simulink model "HIL_model"  (R2020a)
settings: Solver=ode4  StartTime=0.0  StopTime=inf  FixedStep=0.01  RelTol=1e-3
InitFcn:
  | Init_control
values from neighbouring files (symbols this model uses):
  layer1 = double(results{1,1}.layer9)    [load_parameter.m]
  layer2 = double(results{1,1}.layer10)    [load_parameter.m]
  layer3 = double(results{1,1}.layer11)    [load_parameter.m]
  layer4 = double(results{1,1}.layer12)    [load_parameter.m]
  layer5 = double(results{1,1}.layer13)    [load_parameter.m]
  layer6 = double(results{1,1}.layer14)    [load_parameter.m]
  std = sqrt(max(a,0.01))    [load_parameter.m]
undefined symbols (not defined in the file or in its folder): KiPitchAttitude, KiRollAttitude, Kp_RP_ANGLE, MAX_CONTROL_ANGLE_RATE_Y, MAX_CONTROL_ANGLE_RP
libraries: simulink x3, pixhawk_slib_uORB_RW x2, pixhawk_slib_sensors_actuators x2
settings Model: Creator=Steve  LastModifiedBy=NEW
settings SolverCC: AutoInsertRateTranBlk=on
settings DataIOCC: LimitDataPoints=on  SaveFormat=Array  ReturnWorkspaceOutputs=off
settings OptimizationCC: DefaultParameterBehavior=Inlined  LifeSpan=1  MaxStackSize=64  EfficientTunableParamExpr=on
settings DebuggingCC: SolverPrmCheckMsg=warning  AllowSymbolicDim=off  SFUnexpectedBacktrackingDiag=warning  SFNoUnconditionalDefaultTransitionDiag=warning  SFExecutionAtInitializationDiag=none  ArithmeticOperatorsInVariantConditions=warning
settings HardwareCC: ProdBitPerPointer=32  ProdBitPerSizeT=32  ProdBitPerPtrDiffT=32  ProdLargestAtomicInteger=Long  ProdLargestAtomicFloat=Double  ProdWordSize=32  ProdHWDeviceType=ARM Compatible->ARM Cortex
settings ModelReferenceCC: PropagateSignalLabelsOutOfModel=off
settings SFSimCC: SimUseLocalCustomCode=off  MATLABDynamicMemAlloc=off  CustomCodeUndefinedFunction=UseInterfaceOnly
settings RTWCC: SystemTargetFile=ert.tlc  HardwareBoard=Pixhawk PX4  TemplateMakefile=ert_default_tmf  GenerateReport=on  RTWUseLocalCustomCode=off  Toolchain=Pixhawk Toolchain  IncludeHyperlinkInReport=on  LaunchReport=on  GenerateTraceReport=on  GenerateTraceReportSl=on  GenerateTraceReportSf=on  GenerateTraceReportEml=on  GenerateCodeMetricsReport=on
settings CodeAppCC: IgnoreCustomStorageClasses=off  StateflowObjectComments=on
settings ERTTargetCC: CodeReplacementLibrary=GCC ARM Cortex-A9  MultiwordLength=2048  ExtModeTransport=1  ExtModeMexFile=ext_serial_win32_comm  ExtModeMexArgs=/dev/serial  ERTCustomFileTemplate=PX4_codertarget_file_process.tlc  ConvertIfToSwitch=off  SuppressUnreachableDefaultCases=off
settings ConfigComp: CovMetricSettings=dw  CovHtmlReporting=on  CovSaveCumulativeToWorkspaceVar=on  CovSaveSingleToWorkspaceVar=on  CovExternalEMLEnable=off  CovSFcnEnable=off

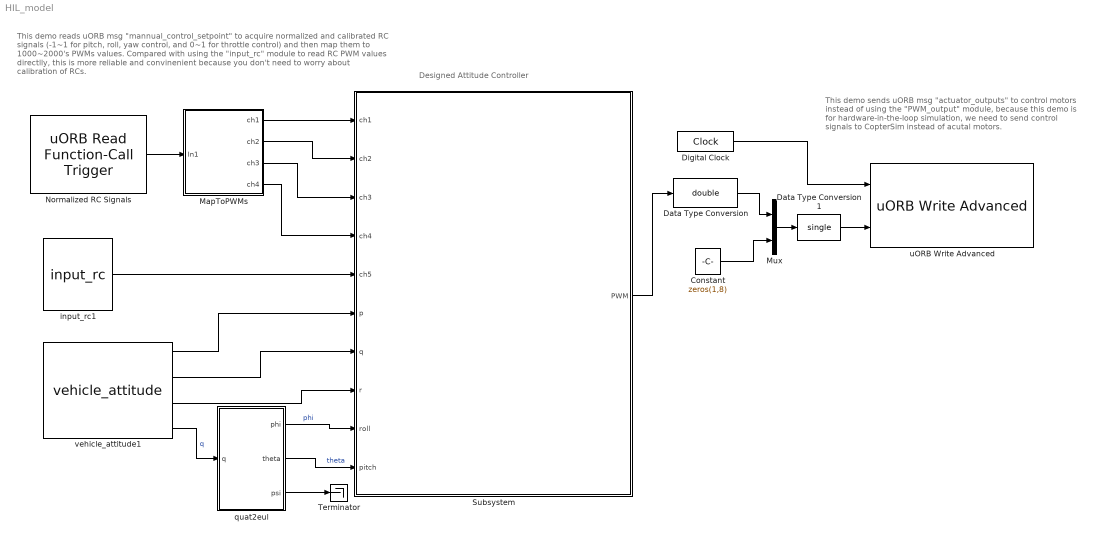
== system HIL_model ==
  note: Designed Attitude Controller
  note: This demo reads uORB msg "mannual_control_setpoint" to acquire normalized and calibrated RC signals (-1~1 for pitch, roll, yaw control, and 0~1 for throttle control) and then map them to 1000~2000's PWMs values.
      | Compared with using the "input_rc" module to read RC PWM values directlly, this is more reliable and convinenient because you don't need to worry about calibration of RCs.
  note: This demo sends uORB msg "actuator_outputs" to control motors instead of using the "PWM_output" module, because this demo is for hardware-in-the-loop simulation, we need to send control signals to CopterSim instead of acutal motors.
  Constant : Constant  Value=zeros(1,8)
  Data Type Conversion : DataTypeConversion  OutDataTypeStr=double
  Data Type Conversion1 : DataTypeConversion  OutDataTypeStr=single
  Digital Clock : DigitalClock  SampleTime=-1
  MapToPWMs : Subsystem
  Mux : Mux  Inputs=2
  Normalized RC Signals : pixhawk_slib_uORB_RW/uORB Read Function-Call Trigger  uORB_Topic_str='manual_control_setpoint'  BusObjVar=Bus: manual_control_setpoint_SL  uORB_Interval=1  AsyncOutput=off  Fcn_call_select=Generate Function Call Signal  TaskName='Task1'  Poll_timeout=100  Ts=-1
      settings: SourceProductName=Pixhawk Target Blocks
  Subsystem : Subsystem
      mask Display: image('./icon/pixhawk.png');
  Terminator : Terminator
  input_rc1 : pixhawk_slib_sensors_actuators/input_rc  Description=|  sampletime=-1  channel1=off  channel2=off  channel3=off  channel4=off  channel5=on  channel6=off  channel7=off  channel8=off  channel9=off  channel10=off  channel11=off  channel12=off  channel13=off  channel14=off  channel15=off  channel16=off  channel17=off  channel18=off  ch_count=off  rssi=off  rc_failsafe=off  rc_lost=off  rc_inputsource=off
      | RC Input Block
      | 
      | This block provides user input control to the model.
      | It uses the input_rc uORB topic.
      | 
      | The user has the ability to choose which channels are available as outputs from this block and also some optional outputs. These include 
      | Channels 1 through 18
      | double data type indicating the PWM value from the controller 
      | measured pulse widths for each of the supported channels 
      | Channel Count 
      | uint32 data type of the number of channels which are detector by the PX4 
      | RC Failsafe 
      | boolean data types indicating that the RC Tx is sending the FailSafe signal (if equipped and properly setup) 
      | explicit failsafe flag: true on TX failure or TX out of range , false otherwise. 
      | Only the true state is reliable, as there are some (PPM) receivers on the market going into failsafe without telling us explicitly. 
      | RC Input Source 
      | Enumeration data type indicating which source the RC input is from. 
      | Valid values are found in the ENUM file: RC_INPUT_SOURCE_ENUM.m 
      |           Enumeration members for class 'RC_INPUT_SOURCE_ENUM':
      |           RCINPUT_SOURCE_UNKNOWN         (0)
      |           RCINPUT_SOURCE_PX4FMU_PPM      (1)
      |           RCINPUT_SOURCE_PX4IO_PPM       (2)
      |           RCINPUT_SOURCE_PX4IO_SPEKTRUM  (3)
      |           RCINPUT_SOURCE_PX4IO_SBUS      (4)
      |           RCINPUT_SOURCE_PX4IO_ST24      (5)
      |           RCINPUT_SOURCE_MAVLINK         (6)
      |           RCINPUT_SOURCE_QURT            (7)
      |           RCINPUT_SOURCE_PX4FMU_SPEKTRUM (8)
      |           RCINPUT_SOURCE_PX4FMU_SBUS     (9)
      |           RCINPUT_SOURCE_PX4FMU_ST24     (10)
      |           RCINPUT_SOURCE_PX4FMU_SUMD     (11)
      |           RCINPUT_SOURCE_PX4FMU_DSM      (12)
      |           RCINPUT_SOURCE_PX4IO_SUMD      (13)
      | 
      | RSSI - Receive signal strength index 
      | receive signal strength indicator (RSSI): < 0: Undefined, 0: no signal, 255: full reception 
      | RC Lost Connection 
      | boolean data type indicating RC receiver connection status 
      | True, if no frame has arrived in the expected time, false otherwise. 
      | True usally means that the receiver has been disconnected, but can also indicate a radio link loss on "stupid" systems. 
      | Will remain false, if a RX with failsafe option continues to transmit frames after a link loss. 
      |   
      | Sample Model: px4demo_input_rc.slx
      settings: SourceProductName=Pixhawk Target Blocks
  quat2eul : MATLAB Function  TreatAsAtomicUnit=on
  uORB Write Advanced : pixhawk_slib_uORB_RW/uORB Write Advanced  Ts=0  uORB_AdvtQueue=on  uORB_FieldEnabledArr="0  0  0  1  0  0  0  0  0  0  0"  uORB_Topic_str=0  uORB_Struct_DT="[1  1  1  1  1]"  BlockInputCount=5  uORB_StructParams="[\"voltage_v\",\"voltage_filtered_v\",\"current_a\",\"current_filtered_a\",\"remaining\"]"  uORB_PortSizes="[1  1  1  1]"  MsgSizeOf=0  MW_update=true
      settings: SourceProductName=Pixhawk Target Blocks
  vehicle_attitude1 : pixhawk_slib_sensors_actuators/vehicle_attitude  sampletime=-1  show_r=on  show_p=on  show_y=on  show_q=on  show_ts=off
      settings: SourceProductName=Pixhawk Target Blocks
  wires:
  quat2eul/1(phi) -> Subsystem/9(roll)  "phi"
  quat2eul/2(theta) -> Subsystem/10(pitch)  "theta"
  vehicle_attitude1/1 -> Subsystem/6(p)
  vehicle_attitude1/2 -> Subsystem/7(q)
  vehicle_attitude1/3 -> Subsystem/8(r)
  Digital Clock/1 -> uORB Write Advanced/1
  Subsystem/1(PWM) -> Data Type Conversion/1
  Constant/1 -> Mux/2
  Mux/1 -> Data Type Conversion1/1
  Data Type Conversion/1 -> Mux/1
  vehicle_attitude1/4 -> quat2eul/1(q)  "q"
  quat2eul/3(psi) -> Terminator/1
  Data Type Conversion1/1 -> uORB Write Advanced/2
  input_rc1/1 -> Subsystem/5(ch5)
  MapToPWMs/4(ch4) -> Subsystem/4(ch4)
  MapToPWMs/3(ch3) -> Subsystem/3(ch3)
  Normalized RC Signals/1 -> MapToPWMs/1(In1)
  MapToPWMs/1(ch1) -> Subsystem/1(ch1)
  MapToPWMs/2(ch2) -> Subsystem/2(ch2)

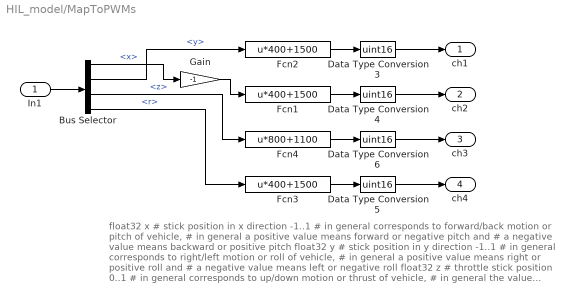
== system HIL_model/MapToPWMs ==
  note: float32 x			 # stick position in x direction -1..1
      | 				 # in general corresponds to forward/back motion or pitch of vehicle,
      | 				 # in general a positive value means forward or negative pitch and
      | 				 # a negative value means backward or positive pitch
      | float32 y			 # stick position in y direction -1..1
      | 				 # in general corresponds to right/left motion or roll of vehicle,
      | 				 # in general a positive value means right or positive roll and
      | 				 # a negative value means left or negative roll
      | float32 z			 # throttle stick position 0..1
      | 				 # in general corresponds to up/down motion or thrust of vehicle,
      | 				 # in general the value corresponds to the demanded throttle by the user,
      | 				 # if the input is used for setting the setpoint of a vertical position
      | 				 # controller any value > 0.5 means up and any value < 0.5 means down
      | float32 r			 # yaw stick/twist position, -1..1
      | 				 # in general corresponds to the righthand rotation around the vertical
      | 				 # (downwards) axis of the vehicle
  In1 : Inport
  Bus Selector : BusSelector  OutputSignals=x,y,z,r
  Data Type Conversion{3..6} (4 alike) : DataTypeConversion  OutDataTypeStr=uint16
  Fcn1 : Fcn  Expr=u*400+1500
  Fcn2 : Fcn  Expr=u*400+1500
  Fcn3 : Fcn  Expr=u*400+1500
  Fcn4 : Fcn  Expr=u*800+1100
  Gain : Gain  Gain=-1
  ch1 : Outport  VectorParamsAs1DForOutWhenUnconnected=off
  ch2 : Outport  Port=2  VectorParamsAs1DForOutWhenUnconnected=off
  ch3 : Outport  Port=3  VectorParamsAs1DForOutWhenUnconnected=off
  ch4 : Outport  Port=4  VectorParamsAs1DForOutWhenUnconnected=off
  wires:
  Bus Selector/2 -> Fcn2/1  "<y>"
  Fcn2/1 -> Data Type Conversion3/1
  Bus Selector/1 -> Gain/1  "<x>"
  In1/1 -> Bus Selector/1
  Bus Selector/3 -> Fcn4/1  "<z>"
  Fcn1/1 -> Data Type Conversion4/1
  Bus Selector/4 -> Fcn3/1  "<r>"
  Data Type Conversion4/1 -> ch2/1
  Data Type Conversion5/1 -> ch4/1
  Data Type Conversion6/1 -> ch3/1
  Fcn4/1 -> Data Type Conversion6/1
  Fcn3/1 -> Data Type Conversion5/1
  Data Type Conversion3/1 -> ch1/1
  Gain/1 -> Fcn1/1

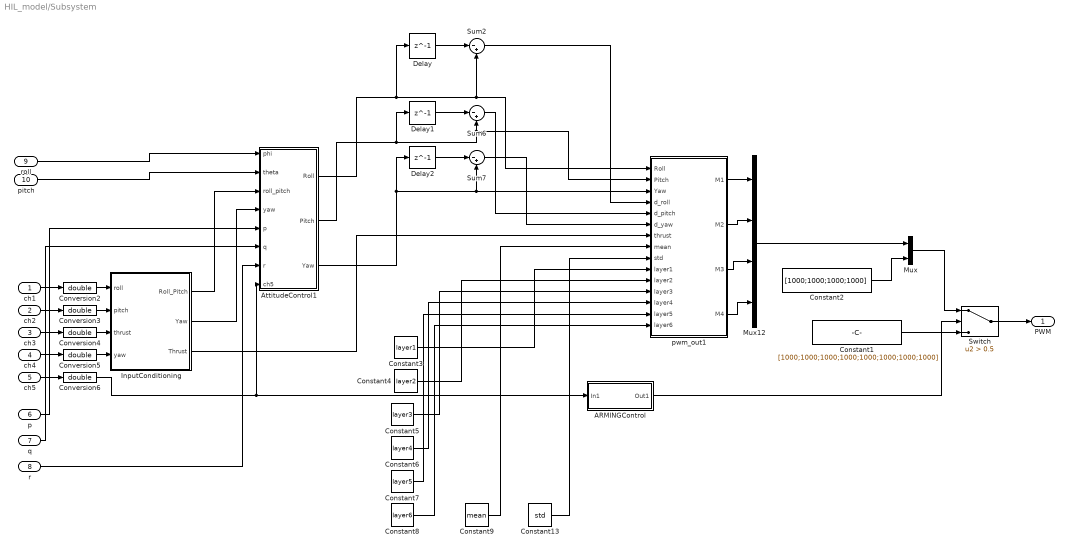
== system HIL_model/Subsystem ==
  ch1 : Inport  OutDataTypeStr=uint16  PortDimensions=1
  ch2 : Inport  Port=2  OutDataTypeStr=uint16  PortDimensions=1
  ch3 : Inport  Port=3  OutDataTypeStr=uint16  PortDimensions=1
  ch4 : Inport  Port=4  OutDataTypeStr=uint16  PortDimensions=1
  ch5 : Inport  Port=5  OutDataTypeStr=uint16  PortDimensions=1  Interpolate=off
  p : Inport  Port=6  PortDimensions=1
  q : Inport  Port=7  PortDimensions=1
  r : Inport  Port=8  PortDimensions=1
  roll : Inport  Port=9  PortDimensions=1
  pitch : Inport  Port=10  PortDimensions=1
  ARMINGControl : Subsystem
  AttitudeControl1 : Subsystem
  Constant1 : Constant  Value=[1000;1000;1000;1000;1000;1000;1000;1000]
  Constant13 : Constant  Value=std
  Constant2 : Constant  Value=[1000;1000;1000;1000]
  Constant3 : Constant  Value=layer1
  Constant4 : Constant  Value=layer2
  Constant5 : Constant  Value=layer3
  Constant6 : Constant  Value=layer4
  Constant7 : Constant  Value=layer5
  Constant8 : Constant  Value=layer6
  Constant9 : Constant  Value=mean
  Conversion{2..6} (5 alike) : DataTypeConversion  OutDataTypeStr=double
  Delay : Delay  DelayLength=1  InitialCondition=0
  Delay1 : Delay  DelayLength=1  InitialCondition=0
  Delay2 : Delay  DelayLength=1  InitialCondition=0
  InputConditioning : Subsystem
  Mux : Mux  Inputs=2
  Mux12 : Mux
  Sum2 : Sum  Inputs=|-+
  Sum6 : Sum  Inputs=|-+
  Sum7 : Sum  Inputs=|-+
  Switch : Switch  Criteria=u2 > Threshold  Threshold=0.5
  pwm_out1 : MATLAB Function  TreatAsAtomicUnit=on
  PWM : Outport  PortDimensions=8  VectorParamsAs1DForOutWhenUnconnected=off
  wires:
  InputConditioning/3(Thrust) -> pwm_out1/7(thrust)
  q/1 -> AttitudeControl1/6(q)
  ARMINGControl/1(Out1) -> Switch/2
  pitch/1 -> AttitudeControl1/2(theta)
  Conversion5/1 -> InputConditioning/4(yaw)
  Mux12/1 -> Mux/1
  pwm_out1/1(M1) -> Mux12/1
  pwm_out1/2(M2) -> Mux12/2
  ch4/1 -> Conversion5/1
  r/1 -> AttitudeControl1/7(r)
  ch2/1 -> Conversion3/1
  ch5/1 -> Conversion6/1
  roll/1 -> AttitudeControl1/1(phi)
  Conversion3/1 -> InputConditioning/2(pitch)
  Conversion4/1 -> InputConditioning/3(thrust)
  Conversion6/1 -> AttitudeControl1/8(ch5), ARMINGControl/1(In1)
  Conversion2/1 -> InputConditioning/1(roll)
  ch1/1 -> Conversion2/1
  pwm_out1/4(M4) -> Mux12/4
  p/1 -> AttitudeControl1/5(p)
  ch3/1 -> Conversion4/1
  InputConditioning/1(Roll_Pitch) -> AttitudeControl1/3(roll_pitch)
  pwm_out1/3(M3) -> Mux12/3
  Constant2/1 -> Mux/2
  InputConditioning/2(Yaw) -> AttitudeControl1/4(yaw)
  Mux/1 -> Switch/1
  Switch/1 -> PWM/1
  Constant1/1 -> Switch/3
  Constant7/1 -> pwm_out1/14(layer5)
  Constant6/1 -> pwm_out1/13(layer4)
  Constant3/1 -> pwm_out1/10(layer1)
  Constant8/1 -> pwm_out1/15(layer6)
  Constant5/1 -> pwm_out1/12(layer3)
  Constant4/1 -> pwm_out1/11(layer2)
  Constant13/1 -> pwm_out1/9(std)
  Constant9/1 -> pwm_out1/8(mean)
  Sum2/1 -> pwm_out1/4(d_roll)
  Sum7/1 -> pwm_out1/6(d_yaw)
  Sum6/1 -> pwm_out1/5(d_pitch)
  Delay/1 -> Sum2/1
  AttitudeControl1/2(Pitch) -> Delay1/1, pwm_out1/2(Pitch), Sum6/2
  AttitudeControl1/1(Roll) -> Delay/1, pwm_out1/1(Roll), Sum2/2
  Delay1/1 -> Sum6/1
  AttitudeControl1/3(Yaw) -> Delay2/1, Sum7/2, pwm_out1/3(Yaw)
  Delay2/1 -> Sum7/1

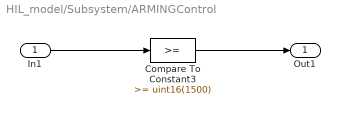
== system HIL_model/Subsystem/ARMINGControl ==
  In1 : Inport
  Compare To Constant3 : simulink/Logic and Bit Operations/Compare To Constant  relop=>=  const=uint16(1500)  OutDataTypeStr=boolean
  Out1 : Outport  VectorParamsAs1DForOutWhenUnconnected=off
  wires:
  Compare To Constant3/1 -> Out1/1
  In1/1 -> Compare To Constant3/1

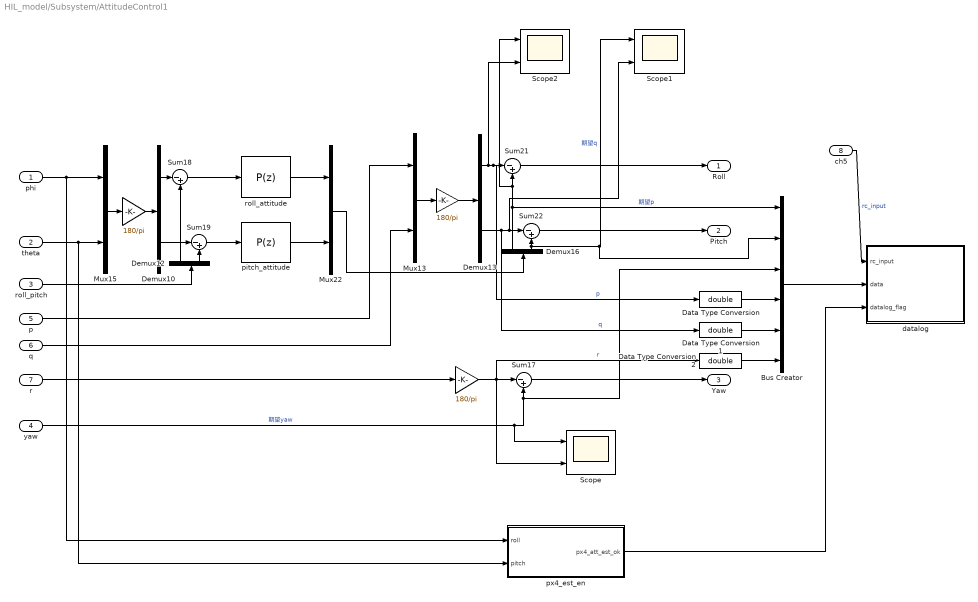
== system HIL_model/Subsystem/AttitudeControl1 ==
  phi : Inport
  theta : Inport  Port=2
  roll_pitch : Inport  Port=3
  yaw : Inport  Port=4
  p : Inport  Port=5
  q : Inport  Port=6
  r : Inport  Port=7
  ch5 : Inport  Port=8
  " " : Gain  Gain=180/pi
  "  " : Gain  Gain=180/pi
  "          " : Gain  Gain=180/pi
  Bus Creator : BusCreator  Inputs=6
  Data Type Conversion : DataTypeConversion  OutDataTypeStr=double
  Data Type Conversion1 : DataTypeConversion  OutDataTypeStr=double
  Data Type Conversion2 : DataTypeConversion  OutDataTypeStr=double
  Demux{10,12..13,16} (4 alike) : Demux  Outputs=2
  Mux13 : Mux  Inputs=2
  Mux15 : Mux  Inputs=2
  Mux22 : Mux  Inputs=2
  Scope : Scope  NumInputPorts=2
  Scope1 : Scope  NumInputPorts=2
  Scope2 : Scope  NumInputPorts=2
  Sum{17..19,21..22} (5 alike) : Sum  Inputs=|-+
  "datalog " : Subsystem
  pitch_attitude : simulink/Continuous/PID Controller  Controller=P  Form=Parallel  TimeDomain=Discrete-time  UseExternalTs=off  SampleTime=-1  IntegratorMethod=Forward Euler  FilterMethod=Forward Euler  ControllerParametersSource=internal  P=Kp_RP_ANGLE  I=KiPitchAttitude  D=0.01  UseFilter=on  N=100  TunerSelectOption=Transfer Function Based (PID Tuner App)  InitialConditionSource=internal  InitialConditionForIntegrator=0  InitialConditionForFilter=0  DifferentiatorICPrevScaledInput=0  ExternalReset=none  TrackingMode=off  Kt=1  LimitOutput=on  UpperSaturationLimit=180  LowerSaturationLimit=-180  LinearizeAsGain=on  AntiWindupMode=back-calculation  Kb=1  POutMin=[]  POutMax=[]  IOutMin=[]  IOutMax=[]  DOutMin=[]  DOutMax=[]  NOutMin=[]  NOutMax=[]  SumOutMin=[]  SumOutMax=[]  SaturationOutMin=[]  SaturationOutMax=[]  PParamMin=[]  PParamMax=[]  IParamMin=[]  IParamMax=[]  DParamMin=[]  DParamMax=[]  NParamMin=[]  NParamMax=[]  KbParamMin=[]  KbParamMax=[]  KtParamMin=[]  KtParamMax=[]  KbOutMin=[]  KbOutMax=[]  KtOutMin=[]  KtOutMax=[]  IntegratorOutMin=[]  IntegratorOutMax=[]  FilterOutMin=[]  FilterOutMax=[]  SumI1OutMin=[]  SumI1OutMax=[]  SumI2OutMin=[]  SumI2OutMax=[]  SumI3OutMin=[]  SumI3OutMax=[]  SumI4OutMin=[]  SumI4OutMax=[]  SumDOutMin=[]  SumDOutMax=[]  DifferentiatorOutMin=[]  DifferentiatorOutMax=[]  FilterDiffOutCoefMin=[]  FilterDiffOutCoefMax=[]  ReciprocalOutMin=[]  ReciprocalOutMax=[]  SumDenOutMin=[]  SumDenOutMax=[]  SumNumOutMin=[]  SumNumOutMax=[]  DivideOutMin=[]  DivideOutMax=[]  UdiffTsProdOutMin=[]  UdiffTsProdOutMax=[]  NTsProdOutMin=[]  NTsProdOutMax=[]  UintegralTsProdOutMin=[]  UintegralTsProdOutMax=[]  UngainTsProdOutMin=[]  UngainTsProdOutMax=[]  IntegratorContinuousStateAttributes=''  IntegratorStateMustResolveToSignalObject=off  IntegratorRTWStateStorageClass=Auto  FilterContinuousStateAttributes=''  FilterStateMustResolveToSignalObject=off  FilterRTWStateStorageClass=Auto  ParallelPVariant=InternalParameters  IdealPVariant=Disabled  IVariant=Disabled  DVariant=Disabled  IntegratorVariant=Disabled  SatVariant=Enabled  AWVariant=Disabled  PCopyVariant=Disabled  TRVariant=Disabled  FdbkBlocksVariant=Forward  IdealPFdbkVariant=Disabled  SatFdbkVariant=Disabled  DerivativeFilterVariant=Disabled  NVariant=Disabled  NCopyVariant=Disabled_SignalSpec  FilterICVariant=Disabled  IntegratorICVariant=Disabled  ExternalResetVariant=Disabled  TRSumVariant=Passthrough  SumFdbkVariant=Disabled  SumVariant=Passthrough_P  TsampFilterVariant=InternalTs  TsampNgainVariant=Passthrough  TsampIntegralVariant=Disabled_SignalSpec
  px4_est_en : MATLAB Function  TreatAsAtomicUnit=on
  roll_attitude : simulink/Continuous/PID Controller  Controller=P  Form=Parallel  TimeDomain=Discrete-time  UseExternalTs=off  SampleTime=-1  IntegratorMethod=Forward Euler  FilterMethod=Forward Euler  ControllerParametersSource=internal  P=Kp_RP_ANGLE  I=KiRollAttitude  D=0.01  UseFilter=on  N=100  TunerSelectOption=Transfer Function Based (PID Tuner App)  InitialConditionSource=internal  InitialConditionForIntegrator=0  InitialConditionForFilter=0  DifferentiatorICPrevScaledInput=0  ExternalReset=none  TrackingMode=off  Kt=1  LimitOutput=on  UpperSaturationLimit=180  LowerSaturationLimit=-180  LinearizeAsGain=on  AntiWindupMode=back-calculation  Kb=1  POutMin=[]  POutMax=[]  IOutMin=[]  IOutMax=[]  DOutMin=[]  DOutMax=[]  NOutMin=[]  NOutMax=[]  SumOutMin=[]  SumOutMax=[]  SaturationOutMin=[]  SaturationOutMax=[]  PParamMin=[]  PParamMax=[]  IParamMin=[]  IParamMax=[]  DParamMin=[]  DParamMax=[]  NParamMin=[]  NParamMax=[]  KbParamMin=[]  KbParamMax=[]  KtParamMin=[]  KtParamMax=[]  KbOutMin=[]  KbOutMax=[]  KtOutMin=[]  KtOutMax=[]  IntegratorOutMin=[]  IntegratorOutMax=[]  FilterOutMin=[]  FilterOutMax=[]  SumI1OutMin=[]  SumI1OutMax=[]  SumI2OutMin=[]  SumI2OutMax=[]  SumI3OutMin=[]  SumI3OutMax=[]  SumI4OutMin=[]  SumI4OutMax=[]  SumDOutMin=[]  SumDOutMax=[]  DifferentiatorOutMin=[]  DifferentiatorOutMax=[]  FilterDiffOutCoefMin=[]  FilterDiffOutCoefMax=[]  ReciprocalOutMin=[]  ReciprocalOutMax=[]  SumDenOutMin=[]  SumDenOutMax=[]  SumNumOutMin=[]  SumNumOutMax=[]  DivideOutMin=[]  DivideOutMax=[]  UdiffTsProdOutMin=[]  UdiffTsProdOutMax=[]  NTsProdOutMin=[]  NTsProdOutMax=[]  UintegralTsProdOutMin=[]  UintegralTsProdOutMax=[]  UngainTsProdOutMin=[]  UngainTsProdOutMax=[]  IntegratorContinuousStateAttributes=''  IntegratorStateMustResolveToSignalObject=off  IntegratorRTWStateStorageClass=Auto  FilterContinuousStateAttributes=''  FilterStateMustResolveToSignalObject=off  FilterRTWStateStorageClass=Auto  ParallelPVariant=InternalParameters  IdealPVariant=Disabled  IVariant=Disabled  DVariant=Disabled  IntegratorVariant=Disabled  SatVariant=Enabled  AWVariant=Disabled  PCopyVariant=Disabled  TRVariant=Disabled  FdbkBlocksVariant=Forward  IdealPFdbkVariant=Disabled  SatFdbkVariant=Disabled  DerivativeFilterVariant=Disabled  NVariant=Disabled  NCopyVariant=Disabled_SignalSpec  FilterICVariant=Disabled  IntegratorICVariant=Disabled  ExternalResetVariant=Disabled  TRSumVariant=Passthrough  SumFdbkVariant=Disabled  SumVariant=Passthrough_P  TsampFilterVariant=InternalTs  TsampNgainVariant=Passthrough  TsampIntegralVariant=Disabled_SignalSpec
  Roll : Outport  VectorParamsAs1DForOutWhenUnconnected=off
  Pitch : Outport  Port=2  VectorParamsAs1DForOutWhenUnconnected=off
  Yaw : Outport  Port=3  VectorParamsAs1DForOutWhenUnconnected=off
  wires:
  r/1 -> "          "/1
  q/1 -> Mux13/2
  Mux22/1 -> Demux16/1
  Sum17/1 -> Yaw/1
  phi/1 -> px4_est_en/1(roll), Mux15/1
  Mux15/1 -> " "/1
  theta/1 -> px4_est_en/2(pitch), Mux15/2
  "          "/1 -> Data Type Conversion2/1, Scope/2, Sum17/1  "r"
  Sum19/1 -> pitch_attitude/1
  pitch_attitude/1 -> Mux22/2
  roll_attitude/1 -> Mux22/1
  Demux16/1 -> Scope2/1, Sum21/2, Bus Creator/1  "期望p"
  yaw/1 -> Scope/1, Bus Creator/3, Sum17/2  "期望yaw"
  roll_pitch/1 -> Demux12/1
  Demux16/2 -> Bus Creator/2, Scope1/1, Sum22/2  "期望q"
  Demux12/1 -> Sum18/2
  Demux12/2 -> Sum19/2
  p/1 -> Mux13/1
  Demux10/1 -> Sum18/1
  Demux10/2 -> Sum19/1
  " "/1 -> Demux10/1
  Sum18/1 -> roll_attitude/1
  Sum22/1 -> Pitch/1
  Mux13/1 -> "  "/1
  Demux13/1 -> Data Type Conversion/1, Sum21/1, Scope2/2  "p"
  Demux13/2 -> Sum22/1, Scope1/2, Data Type Conversion1/1  "q"
  "  "/1 -> Demux13/1
  Sum21/1 -> Roll/1
  px4_est_en/1(px4_att_est_ok) -> "datalog "/3(datalog_flag)
  ch5/1 -> "datalog "/1(rc_input)  "rc_input"
  Bus Creator/1 -> "datalog "/2(data)
  Data Type Conversion/1 -> Bus Creator/4
  Data Type Conversion1/1 -> Bus Creator/5
  Data Type Conversion2/1 -> Bus Creator/6

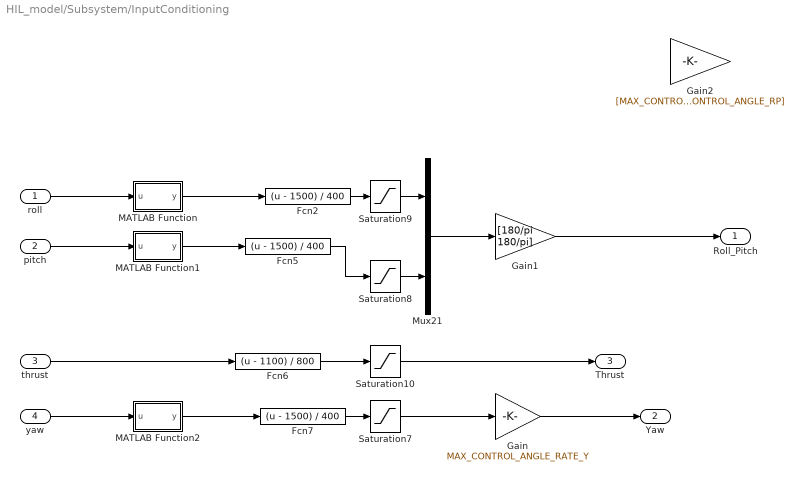
== system HIL_model/Subsystem/InputConditioning ==
  roll : Inport
  pitch : Inport  Port=2
  thrust : Inport  Port=3
  yaw : Inport  Port=4
  Fcn2 : Fcn  Expr=(u - 1500) / 400
  Fcn5 : Fcn  Expr=(u - 1500) / 400
  Fcn6 : Fcn  Expr=(u - 1100) / 800
  Fcn7 : Fcn  Expr=(u - 1500) / 400
  Gain : Gain  Gain=MAX_CONTROL_ANGLE_RATE_Y
  Gain1 : Gain  Gain=[180/pi 180/pi]  OutDataTypeStr=Inherit: Inherit via back propagation
  Gain2 : Gain  Gain=[MAX_CONTROL_ANGLE_RP MAX_CONTROL_ANGLE_RP]  OutDataTypeStr=Inherit: Inherit via back propagation
  MATLAB Function : MATLAB Function  TreatAsAtomicUnit=on
  MATLAB Function1 : MATLAB Function  TreatAsAtomicUnit=on
  MATLAB Function2 : MATLAB Function  TreatAsAtomicUnit=on
  Mux21 : Mux  Inputs=2
  Saturation10 : Saturate  UpperLimit=1  LowerLimit=0
  Saturation7 : Saturate  UpperLimit=1  LowerLimit=-1
  Saturation8 : Saturate  UpperLimit=1  LowerLimit=-1
  Saturation9 : Saturate  UpperLimit=1  LowerLimit=-1
  Roll_Pitch : Outport  VectorParamsAs1DForOutWhenUnconnected=off
  Yaw : Outport  Port=2  VectorParamsAs1DForOutWhenUnconnected=off
  Thrust : Outport  Port=3  VectorParamsAs1DForOutWhenUnconnected=off
  wires:
  Saturation10/1 -> Thrust/1
  Saturation7/1 -> Gain/1
  Gain1/1 -> Roll_Pitch/1
  Mux21/1 -> Gain1/1
  Saturation8/1 -> Mux21/2
  Fcn6/1 -> Saturation10/1
  Fcn2/1 -> Saturation9/1
  Fcn5/1 -> Saturation8/1
  Saturation9/1 -> Mux21/1
  Fcn7/1 -> Saturation7/1
  pitch/1 -> MATLAB Function1/1(u)
  MATLAB Function2/1(y) -> Fcn7/1
  thrust/1 -> Fcn6/1
  roll/1 -> MATLAB Function/1(u)
  MATLAB Function1/1(y) -> Fcn5/1
  MATLAB Function/1(y) -> Fcn2/1
  yaw/1 -> MATLAB Function2/1(u)
  Gain/1 -> Yaw/1

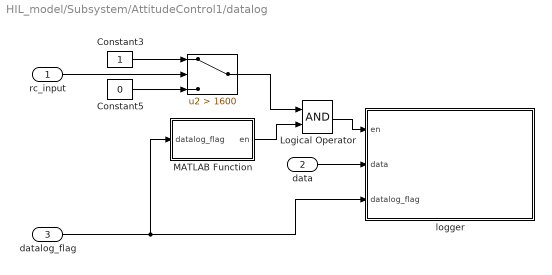
== system HIL_model/Subsystem/AttitudeControl1/datalog  ==
  rc_input : Inport
  data : Inport  Port=2
  datalog_flag : Inport  Port=3
  " " : Switch  Criteria=u2 > Threshold  Threshold=1600
  Constant3 : Constant
  Constant5 : Constant  Value=0
  Logical Operator : Logic  AllPortsSameDT=off  OutDataTypeStr=boolean
  MATLAB Function : MATLAB Function  TreatAsAtomicUnit=on
  logger : Subsystem  mask(Binary Logger){logfile=/fs/microsd/log/e4, cacheflag=off, numRecs=60000}
      mask prompts: cacheflag "Cache in Memory"; numRecs "Max Record Count"
      mask help:
      | Log a vector of data to a file on the SD card
      |
      | If Cache in Memory is on data is written when en goes low or when max number of records specified is reached.
      | Otherwise Max Number of Records is used to indicate when to performa an fflush out to file.
      mask init:
      | logname=uint8(logfile);
      mask Help: eval('pixhawk.internal.doc(''binary_logger_Block.html'')');
      mask Display:
      | fprintf(get_param(gcb,'logfile'))
      | port_label('input',1,'en')
      | port_label('input',2,'data')
      | port_label('input',3,'datalog_flag')
  wires:
  rc_input/1 -> " "/2
  data/1 -> logger/2(data)
  datalog_flag/1 -> logger/3(datalog_flag), MATLAB Function/1(datalog_flag)
  Constant3/1 -> " "/1
  Constant5/1 -> " "/3
  " "/1 -> Logical Operator/1
  MATLAB Function/1(en) -> Logical Operator/2
  Logical Operator/1 -> logger/1(en)

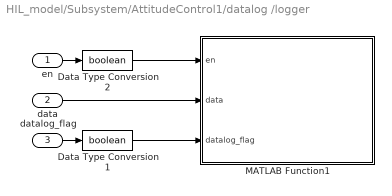
== system HIL_model/Subsystem/AttitudeControl1/datalog /logger ==
  en : Inport
  data : Inport  Port=2
  datalog_flag : Inport  Port=3
  Data Type Conversion1 : DataTypeConversion  OutDataTypeStr=boolean
  Data Type Conversion2 : DataTypeConversion  OutDataTypeStr=boolean
  MATLAB Function1 : MATLAB Function  TreatAsAtomicUnit=on
  wires:
  data/1 -> MATLAB Function1/2(data)
  Data Type Conversion2/1 -> MATLAB Function1/1(en)
  en/1 -> Data Type Conversion2/1
  datalog_flag/1 -> Data Type Conversion1/1
  Data Type Conversion1/1 -> MATLAB Function1/3(datalog_flag)

== matlab function HIL_model/quat2eul ==
  data: q input; phi output; theta output; psi output
function [phi,theta,psi] = quat2eul(q)
% Conversion from Quaternion to Euler angles based on the PX4 Firmware
% v1.6.5 release.
% 
% Quaternion -> DCM -> Euler Angles
% INPUT:
%   q: Quaternion vector of the format: (a + bi + cj + dk)
% OUTPUT:
%   [phi,theta,psi]: Euler angles in radians.
% 
 
    a = q(1);
    b = q(2);
    c = q(3);
    d = q(4);

    aSq = a*a;
    bSq = b*b;
    cSq = c*c;
    dSq = d*d;

    d_pi2 = pi/2;

    % quaternion_to_dcm
    dcm00 = aSq + bSq - cSq - dSq;
    % dcm01 = 2*(b*c - a*d);
    dcm02 = 2*(a*c + b*d);
    dcm10 = 2*(b*c + a*d);
    % dcm11 = aSq - bSq + cSq - dSq;
    dcm12 = 2*(c*d - a*b);
    dcm20 = 2*(b*d - a*c);
    dcm21 = 2*(a*b + c*d);
    dcm22 = aSq - bSq - cSq + dSq;

    % dcm_to_euler
    theta = asin(-dcm20);
    if abs(theta - d_pi2) < 1.0e-3
        phi = single(0.0);
        psi = atan2(dcm12, dcm02);
    elseif abs(theta + d_pi2) < 1.0e-3
        phi = single(0.0);
        psi = atan2(-dcm12, -dcm02);
    else
        phi = atan2(dcm21, dcm22);
        psi = atan2(dcm10, dcm00);
    end

end

== matlab function HIL_model/Subsystem/InputConditioning/MATLAB Function ==
  data: u input; y output
function y = fcn(u)

 if(u>1550)
    y=u;
 else
     if(u<1450)
     y=u;
     else
         y=1500;
     end
 end

== matlab function HIL_model/Subsystem/InputConditioning/MATLAB Function1 ==
  data: u input; y output
function y = fcn(u)

 if(u>1550)
    y=u;
 else
     if(u<1450)
     y=u;
     else
         y=1500;
     end
 end

== matlab function HIL_model/Subsystem/InputConditioning/MATLAB Function2 ==
  data: u input; y output
function y = fcn(u)

 if(u>1550)
    y=u;
 else
     if(u<1450)
     y=u;
     else
         y=1500;
     end
 end

== matlab function HIL_model/Subsystem/AttitudeControl1/datalog /MATLAB Function ==
  data: datalog_flag input; en output
function en = fcn(datalog_flag)

persistent count;
if isempty(count)
    count = 0;
end

if datalog_flag
    count = count + 1;
end
if count > 60000
    en = false;
    count = 0;
else
    en = true;
end

== matlab function HIL_model/Subsystem/AttitudeControl1/datalog /logger/MATLAB Function1 ==
  data: en input boolean; data input; datalog_flag input boolean; logname parameter uint8; cacheflag parameter boolean; numRecs parameter uint32
%% Binary Logger
% Note: All data needs to be of the same type (e.g. double)
% Header information format:
%           String "MWLOGV##"
%           Time/Date 4 bytes (time())
%           Number of Signals per record Logged 1 byte (256 max)
%           Data Type of Signals Logged  1 byte (1-10)
%           Number of bytes per record 2 bytes (65535 max)
% This does NOT include the number of data sets logged.  
% i.e. The Reader is responsible for reading until EOF.
% MathWorks Pilot Engineering 2015
% Steve Kuznicki
function binary_logger(en, data, datalog_flag, logname, cacheflag, numRecs)
%#codegen
    persistent fp isflushed isopen count lognumstr elem_size vect_size
    coder.cinclude('<stdio.h>');
    coder.cinclude('<time.h>');
    
    if isempty(count)
        count = uint32(0);
        lognumstr = 65;
        isopen = false;
        fp = coder.opaque('FILE*', 'NULL');
        isflushed = false;
        elem_size = uint16(1);
        vect_size = coder.const(uint8(numel(data)));
        if cacheflag == true
            %datastored = zeros(numRecs*uint32(coder.const(numel(data))), 1, 'like', data);
        end
    end

    if (en)
        if isopen == false
            [elsize, eltype] = get_elem_size(data);
            elem_size = coder.const(uint16(elsize));
            elem_type = coder.const(uint8(eltype));
            vect_size = coder.const(uint8(numel(data)));
            coder.ceval('printf',['OPENING file %s vect_size %d elem_size %d numRecs %d %c' uint8(0)], ...
                [logname, '_', char(lognumstr), '.bin', int8(0)], uint32(vect_size), uint32(elem_size), uint32(numRecs), uint8(10));
            fp = coder.ceval('fopen', [logname, '_', char(lognumstr), '.bin', int8(0)], ['wb', int8(0)]);
            lognumstr = lognumstr + 1;
            isflushed = false;
            count = uint32(0);
            isopen = true;
            % Write header information here
            % header token + version
            mlStrVer = 'MWLOGV01';
            coder.ceval('fwrite', coder.rref(mlStrVer), uint32(1), length(mlStrVer), fp);
            % date/time
            tm = uint32(0);
            tmptr = uint32(0);
            tm = coder.ceval('time',coder.wref(tmptr));
            coder.ceval('fwrite', coder.rref(tm), uint32(4), uint32(1), fp);
            % number of elements in each record
            coder.ceval('fwrite', coder.rref(vect_size), uint32(1), uint32(1), fp);
            % data type of the elements
            coder.ceval('fwrite', coder.rref(elem_type), uint32(1), uint32(1), fp);
            % size of each record in bytes
            recSize = elem_size * uint16(vect_size);
            coder.ceval('fwrite', coder.rref(recSize), uint32(2), uint32(1), fp);
        end
        % cache data in memory or use fwrite
        if cacheflag == true
            addr = (count*uint32(vect_size))+1;
            for idx = 1:vect_size
                %datastored(addr) = data(idx);
                addr = addr + 1;
            end
            count = count + uint32(1);
        else
            if  datalog_flag
                coder.ceval('fwrite', coder.rref(data), elem_size, vect_size, fp);
                count = count + uint32(1);
            end
        end
        
        % check for data count limit
        if count >= numRecs
            if cacheflag
                for idx = 1:count*uint32(vect_size)
                    %coder.ceval('fwrite', coder.rref(datastored(idx)), elem_size, uint32(1), fp);
                end
            end
            coder.ceval('fflush', fp);
            isflushed = false;
            count = uint32(0);
        end
    else
        if isopen == true
            if ~isflushed 
                coder.ceval('printf',['CLOSING file. count = %d %c' uint8(0)], uint32(count), uint8(10));
                if cacheflag
                    count = count + uint32(1);
                    for idx = 1:count*uint32(vect_size)
                        %coder.ceval('fwrite', coder.rref(datastored(idx)), elem_size, uint32(1), fp);
                    end
                end
                coder.ceval('fflush', fp);
                isflushed = true;
            end
            coder.ceval('fclose', fp);
        end
        isopen = false;
        count = uint32(0);
    end
end

% return the size of the element in bytes
function [elem_size, dtype] = get_elem_size(data)
    switch(class(data))
        case 'double'
            elem_size = 8;
            dtype = 1;
        case 'single'
            elem_size = 4;
            dtype = 2;
        case 'int32'
            elem_size = 4;
            dtype = 3;
        case 'uint32'
            elem_size = 4;
            dtype = 4;
        case 'int16'
            elem_size = 2;
            dtype = 5;
        case 'uint16'
            elem_size = 2;
            dtype = 6;
        case 'int8'
            elem_size = 1;
            dtype = 7;
        case 'uint8'
            elem_size = 1;
            dtype = 8;
        case 'logical'
            elem_size = 1;
            dtype = 9;
        case 'embedded.fi'
            nt = numerictype(data);
            elem_size = 2^ceil(log2(ceil(nt.WordLength / 8)));
            dtype = 10;
    end
    if ~isreal(data)
        elem_size = elem_size*2;
    end
    
    elem_size = uint16(elem_size);
    dtype = uint8(dtype);
end

== matlab function HIL_model/Subsystem/AttitudeControl1/px4_est_en ==
  data: roll input; px4_att_est_ok output; pitch input
function px4_att_est_ok = px4_est_en(roll, pitch)

if abs(roll) < 0.000001 && abs(pitch) < 0.000001
    px4_att_est_ok = false;
else
    px4_att_est_ok = true;
end

== matlab function HIL_model/Subsystem/pwm_out1 ==
  data: Roll input; M1 output; Pitch input; Yaw input; d_roll input; M2 output; M3 output; M4 output; d_pitch input; d_yaw input; thrust input; mean input; std input; layer1 input; layer2 input; layer3 input; layer4 input; layer5 input; layer6 input
function [M1, M2, M3, M4] = motor_mixer(Roll, Pitch, Yaw,d_roll, d_pitch, d_yaw, thrust, mean, std,layer1,layer2,layer3,layer4,layer5,layer6)


ob = [Roll, Pitch, Yaw,d_roll, d_pitch, d_yaw];
ob = (ob-reshape(mean,1,6))./reshape(std,1,6);
ob = max(ob,[-5.0,-5.0,-5.0,-5.0,-5.0,-5.0]);
ob = min(ob, [5.0,5.0,5.0,5.0,5.0,5.0]);
layer_1 = tanh(ob * layer1 + reshape(layer2, 1, 32));
layer_2 = tanh(layer_1 * layer3 + reshape(layer4, 1, 32));
output = layer_2 * layer5 + reshape(layer6,1,4);

%layer_1 = tanh(ob * layer1 + reshape(layer2, 1, 64));
%layer_2 = tanh(layer_1 * layer3 + reshape(layer4, 1, 64));
%output = layer_2 * layer5 + reshape(layer6,1,4);

u = output;
for i = 1:4
    if output(i)>1
        output(i)=1;
    end
    if output(i)<-1
        output(i) = -1;
    end
    output(i) = (output(i)+1)/2;
end
%O1 = u(1);
%O2 = u(2);
%O3 = u(3);
%O4 = u(4);
pwm = 500*output+1000*thrust + 1000;
M1 = ( pwm(1)) ;
M2 = ( pwm(4)) ;              
M3 = ( pwm(3)) ;
M4 = ( pwm(2)) ;


% Quad XROLL （根据QP里面的叉字形结构的文字）
% M1 = ((Pitch+ Yaw)+Thrust-Roll) * 1000 + idle_PWM;
 %M2 = ((Pitch - Yaw)+Thrust+Roll) * 1000 + idle_PWM;
 %M3 = ((Roll +Yaw) + Thrust-Pitch) * 1000 + idle_PWM;
 %M4 = ((-Roll - Pitch-Yaw) + Thrust) * 1000 + idle_PWM;
% M5 = 1000;
% M6 = 1000;
% M7 = 1000;
% M8 = 1000;
%qp上实际的输出
%M1 = (Thrust+Pitch-Roll+Yaw) * 1000 + idle_PWM;
 %M2 = (Thrust-Pitch +Roll+Yaw) * 1000 + idle_PWM;
 %M3 = ( Thrust+Roll+Pitch-Yaw) * 1000 + idle_PWM;
 %M4 = (Thrust-Roll- Pitch -Yaw) * 1000 + idle_PWM;
% Quad +
 %M1 = ((Pitch - Yaw) * Thrust / 2 + Thrust) * 1000 + idle_PWM;
 %M2 = ((-Roll + Yaw) * Thrust / 2 + Thrust) * 1000 + idle_PWM;
% M3 = ((-Pitch - Yaw) * Thrust / 2 + Thrust) * 1000 + idle_PWM;
 %M4 = ((Roll + Yaw) * Thrust / 2 + Thrust) * 1000 + idle_PWM;
% M5 = 1000;
% M6 = 1000;
% M7 = 1000;
% M8 = 1000;

% Hex X
% M1 = ((Pitch + Roll / 2 - Yaw) * Thrust / 2 + Thrust) * 1000 + idle_PWM;
% M2 = ((Pitch - Roll / 2 + Yaw) * Thrust / 2 + Thrust) * 1000 + idle_PWM;
% M3 = ((-Roll - Yaw) * Thrust / 2 + Thrust) * 1000 + idle_PWM;
% M4 = ((-Pitch - Roll / 2 + Yaw) * Thrust / 2 + Thrust) * 1000 + idle_PWM;
% M5 = ((-Pitch + Roll / 2 - Yaw) * Thrust / 2 + Thrust) * 1000 + idle_PWM;
% M6 = ((Roll + Yaw) * Thrust / 2 + Thrust) * 1000 + idle_PWM;
% M7 = 1000;
% M8 = 1000;

% Hex X (From Adam)
%M1 = uint16(single(((-Roll - Yaw) * Thrust / 3 + Thrust) * single(1000))) + idle_PWM;
%M2 = uint16(single(((Roll + Yaw) * Thrust / 3 + Thrust) * single(1000))) + idle_PWM;
%M3 = uint16(single(((Pitch + (Roll / 2) - Yaw) * Thrust / 3 + Thrust) * single(1000))) + idle_PWM;
%M4 = uint16(single(((-Pitch - (Roll / 2) + Yaw) * Thrust / 3 + Thrust) * single(1000))) + idle_PWM;
%M5 = uint16(single(((Pitch - (Roll / 2) + Yaw) * Thrust / 3 + Thrust) * single(1000))) + idle_PWM;
%M6 = uint16(single(((-Pitch + (Roll / 2) - Yaw) * Thrust / 3 + Thrust) * single(1000))) + idle_PWM;

% Hex X (Version 2)
% Roll/Yaw
% M1 = ((-Roll - Yaw) * Thrust / 2 + Thrust) * 1000 + idle_PWM;
% M2 = ((Roll + Yaw) * Thrust / 2 + Thrust) * 1000 + idle_PWM;
% % + Pitch/Roll
% M6 = ((Pitch + Roll / 2 - Yaw) * Thrust / 2 + Thrust) * 1000 + idle_PWM;
% M4 = ((Pitch - Roll / 2 + Yaw) * Thrust / 2 + Thrust) * 1000 + idle_PWM;
% % - Pitch/Roll
% M5 = ((-Pitch - Roll / 2 + Yaw) * Thrust / 2 + Thrust) * 1000 + idle_PWM;
% M3 = ((-Pitch + Roll / 2 - Yaw) * Thrust / 2 + Thrust) * 1000 + idle_PWM;
